simulink model "CSTR2"  (Simulink 3.00)
settings: Solver=ode45  StartTime=0.0  StopTime=1000.0  RelTol=1e-3
settings Model: LastModifiedBy=Administrator

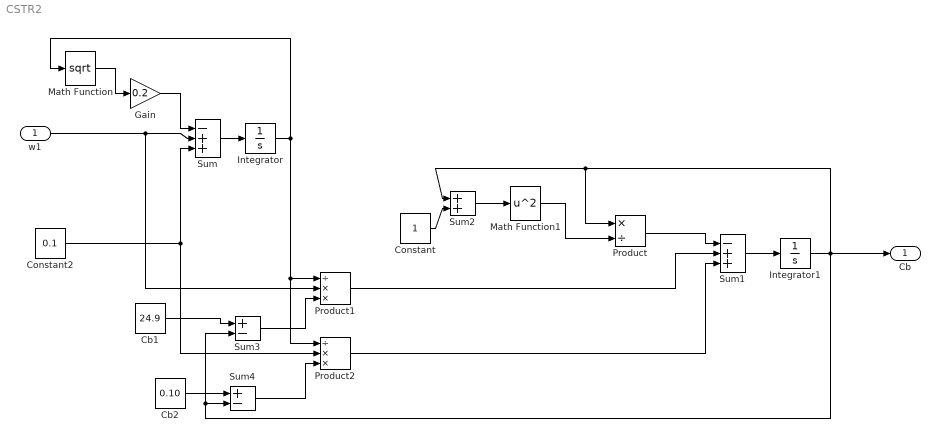
== system CSTR2 ==
  w1 : Inport  Port=1  PortWidth=-1  SampleTime=-1  DataType=auto
      settings: SignalType=auto
  Cb1 : Constant  Value=24.9
  Cb2 : Constant  Value=0.10
  Constant : Constant  Value=1
  Constant2 : Constant  Value=0.1
  Gain : Gain  Gain=0.2  SaturateOnIntegerOverflow=on
  Integrator : Integrator  ExternalReset=none  InitialConditionSource=internal  InitialCondition=30  LimitOutput=on  UpperSaturationLimit=inf  LowerSaturationLimit=1  ShowSaturationPort=off  ShowStatePort=off  AbsoluteTolerance=auto
  Integrator1 : Integrator  ExternalReset=none  InitialConditionSource=internal  InitialCondition=22  LimitOutput=off  UpperSaturationLimit=inf  LowerSaturationLimit=-inf  ShowSaturationPort=off  ShowStatePort=off  AbsoluteTolerance=auto
  Math Function : Math  Operator=sqrt  OutputSignalType=auto
  Math Function1 : Math  Operator=square  OutputSignalType=auto
  Product : Product  Inputs=*/  SaturateOnIntegerOverflow=on
  Product1 : Product  Inputs=/**  SaturateOnIntegerOverflow=on
  Product2 : Product  Inputs=/**  SaturateOnIntegerOverflow=on
  Sum : Sum  Inputs=-++  SaturateOnIntegerOverflow=on
  Sum1 : Sum  Inputs=-++  SaturateOnIntegerOverflow=on
  Sum2 : Sum  Inputs=++  SaturateOnIntegerOverflow=on
  Sum3 : Sum  Inputs=+-  SaturateOnIntegerOverflow=on
  Sum4 : Sum  Inputs=+-  SaturateOnIntegerOverflow=on
  Cb : Outport  Port=1
  wires:
  Sum/1 -> Integrator/1
  Gain/1 -> Sum/1
  Math Function/1 -> Gain/1
  Integrator/1 -> Math Function/1, Product1/1, Product2/1
  Cb1/1 -> Sum3/1
  Cb2/1 -> Sum4/1
  Sum3/1 -> Product1/3
  Sum4/1 -> Product2/3
  Constant/1 -> Sum2/2
  Sum2/1 -> Math Function1/1
  Sum1/1 -> Integrator1/1
  Math Function1/1 -> Product/2
  Product/1 -> Sum1/1
  Product1/1 -> Sum1/2
  Product2/1 -> Sum1/3
  w1/1 -> Sum/2, Product1/2
  Constant2/1 -> Sum/3, Product2/2
  Integrator1/1 -> Sum3/2, Sum4/2, Sum2/1, Product/1, Cb/1
